simulink model "openMHA_test_dualport"  (R2020a)
settings: Solver=VariableStepAuto  StartTime=0.0  StopTime=stop_time  RelTol=1e-3
InitFcn:
  | test_dualport_init
StopFcn:
  | test_dualport_stop
libraries: dspsrcs4 x5, FPGA_Open_Speech_Tools x1
settings Model: Creator=t96f346  LastModifiedBy=t96f346

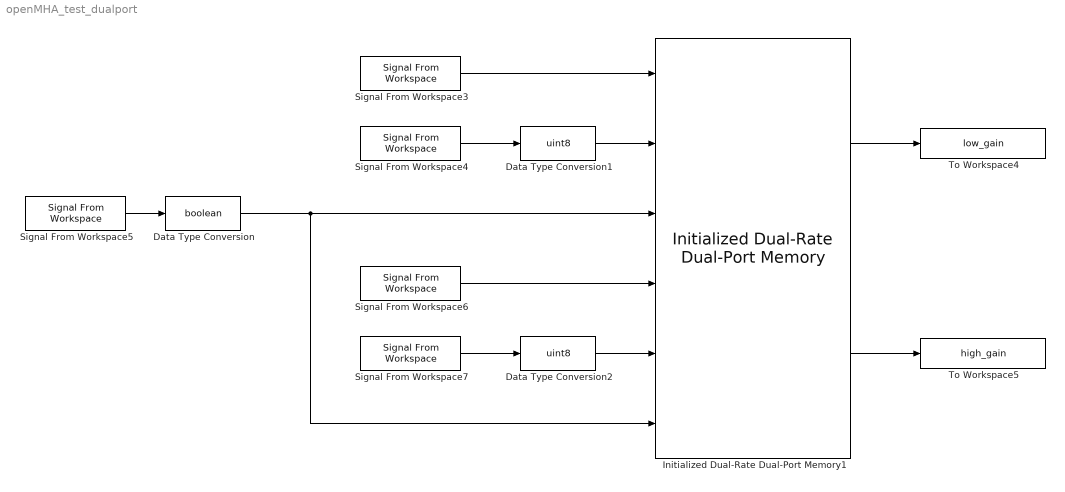
== system openMHA_test_dualport ==
  Data Type Conversion : DataTypeConversion  OutDataTypeStr=boolean
  Data Type Conversion1 : DataTypeConversion  OutDataTypeStr=uint8
  Data Type Conversion2 : DataTypeConversion  OutDataTypeStr=uint8
  Initialized Dual-Rate Dual-Port Memory1 : FPGA_Open_Speech_Tools/Initialized Dual-Rate Dual-Port Memory  ram_size=8  Table_Init=tableInit
  Signal From Workspace3 : dspsrcs4/Signal From Workspace  X=vy_new_gain_low  Ts=1  nsamps=1  OutputAfterFinalValue=Setting to zero  ignoreOrWarnInputAndFrameLengths=off  OutputFrames=off
  Signal From Workspace4 : dspsrcs4/Signal From Workspace  X=vy_address_low  Ts=1  nsamps=1  OutputAfterFinalValue=Setting to zero  ignoreOrWarnInputAndFrameLengths=off  OutputFrames=off
  Signal From Workspace5 : dspsrcs4/Signal From Workspace  X=vy_write_en  Ts=1  nsamps=1  OutputAfterFinalValue=Setting to zero  ignoreOrWarnInputAndFrameLengths=off  OutputFrames=off
  Signal From Workspace6 : dspsrcs4/Signal From Workspace  X=vy_new_gain_high  Ts=1  nsamps=1  OutputAfterFinalValue=Setting to zero  ignoreOrWarnInputAndFrameLengths=off  OutputFrames=off
  Signal From Workspace7 : dspsrcs4/Signal From Workspace  X=vy_address_high  Ts=1  nsamps=1  OutputAfterFinalValue=Setting to zero  ignoreOrWarnInputAndFrameLengths=off  OutputFrames=off
  To Workspace4 : ToWorkspace  VariableName=low_gain  SampleTime=-1
      settings: Save2DSignal=2-D array (concatenate along first dimension)
  To Workspace5 : ToWorkspace  VariableName=high_gain  SampleTime=-1
      settings: Save2DSignal=2-D array (concatenate along first dimension)
  wires:
  Signal From Workspace3/1 -> Initialized Dual-Rate Dual-Port Memory1/1
  Signal From Workspace4/1 -> Data Type Conversion1/1
  Signal From Workspace6/1 -> Initialized Dual-Rate Dual-Port Memory1/4
  Signal From Workspace7/1 -> Data Type Conversion2/1
  Signal From Workspace5/1 -> Data Type Conversion/1
  Initialized Dual-Rate Dual-Port Memory1/1 -> To Workspace4/1
  Initialized Dual-Rate Dual-Port Memory1/2 -> To Workspace5/1
  Data Type Conversion/1 -> Initialized Dual-Rate Dual-Port Memory1/3, Initialized Dual-Rate Dual-Port Memory1/6
  Data Type Conversion1/1 -> Initialized Dual-Rate Dual-Port Memory1/2
  Data Type Conversion2/1 -> Initialized Dual-Rate Dual-Port Memory1/5
